simulink model "mymodel_lilio"  (R2017a)
settings: Solver=FixedStepAuto  StartTime=0  StopTime=100  FixedStep=0.05  RelTol=1e-3
settings Model: Creator=bsolv  LastModifiedBy=bsolv

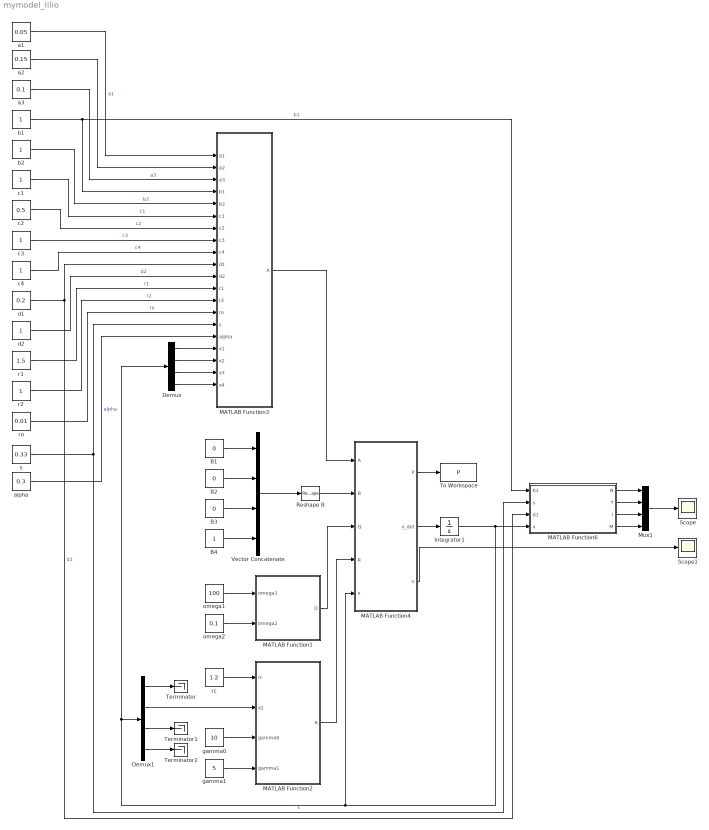
== system mymodel_lilio ==
  B1 : Constant  Value=0
  B2 : Constant  Value=0
  B3 : Constant  Value=0
  B4 : Constant
  Demux : Demux
  Demux1 : Demux
  Integrator1 : Integrator  InitialCondition=[1-1;0.2;0.15-1.65;0]
  MATLAB Function1 : MATLAB Function  TreatAsAtomicUnit=on
  MATLAB Function2 : MATLAB Function  TreatAsAtomicUnit=on
  MATLAB Function3 : MATLAB Function  TreatAsAtomicUnit=on
  MATLAB Function4 : MATLAB Function  TreatAsAtomicUnit=on
  MATLAB Function6 : MATLAB Function  TreatAsAtomicUnit=on
  Mux1 : Mux
  Reshape B : Reshape  OutputDimensionality=Column vector (2-D)
  Scope : Scope
  Scope1 : Scope
  Terminator : Terminator
  Terminator1 : Terminator
  Terminator2 : Terminator
  To Workspace : ToWorkspace  VariableName=P  SampleTime=1
  Vector Concatenate : Concatenate  NumInputs=4
  a1 : Constant  Value=0.05
  a2 : Constant  Value=0.15
  a3 : Constant  Value=0.1
  alpha : Constant  Value=0.3
  b1 : Constant
  b2 : Constant
  c1 : Constant
  c2 : Constant  Value=0.5
  c3 : Constant
  c4 : Constant
  d1 : Constant  Value=0.2
  d2 : Constant
  gamma0 : Constant  Value=10
  gamma1 : Constant  Value=5
  omega1 : Constant  Value=100
  omega2 : Constant  Value=0.1
  r1 : Constant  Value=1.5
  r2 : Constant
  rc : Constant  Value=1.2
  ro : Constant  Value=0.01
  s : Constant  Value=0.33
  wires:
  omega2/1 -> MATLAB Function1/2(omega2)
  omega1/1 -> MATLAB Function1/1(omega1)
  rc/1 -> MATLAB Function2/1(rc)
  gamma0/1 -> MATLAB Function2/3(gamma0)
  B1/1 -> Vector Concatenate/1
  B2/1 -> Vector Concatenate/2
  B3/1 -> Vector Concatenate/3
  B4/1 -> Vector Concatenate/4
  Vector Concatenate/1 -> Reshape B/1
  MATLAB Function3/1(A) -> MATLAB Function4/1(A)
  Reshape B/1 -> MATLAB Function4/2(B)
  MATLAB Function1/1(Q) -> MATLAB Function4/3(Q)
  MATLAB Function2/1(R) -> MATLAB Function4/4(R)
  Demux/1 -> MATLAB Function3/17(x1)
  Demux/2 -> MATLAB Function3/18(x2)
  Demux/3 -> MATLAB Function3/19(x3)
  Demux/4 -> MATLAB Function3/20(x4)
  a1/1 -> MATLAB Function3/1(a1)  "a1"
  a2/1 -> MATLAB Function3/2(a2)
  a3/1 -> MATLAB Function3/3(a3)  "a3"
  b1/1 -> MATLAB Function6/1(b1), MATLAB Function3/4(b1)  "b1"
  b2/1 -> MATLAB Function3/5(b2)  "b2"
  c1/1 -> MATLAB Function3/6(c1)  "c1"
  c2/1 -> MATLAB Function3/7(c2)  "c2"
  c3/1 -> MATLAB Function3/8(c3)  "c3"
  c4/1 -> MATLAB Function3/9(c4)  "c4"
  d1/1 -> MATLAB Function3/10(d1), MATLAB Function6/3(d1)  "d1"
  d2/1 -> MATLAB Function3/11(d2)  "d2"
  r1/1 -> MATLAB Function3/12(r1)  "r1"
  r2/1 -> MATLAB Function3/13(r2)  "r2"
  s/1 -> MATLAB Function3/15(s), MATLAB Function6/2(s)  "s"
  ro/1 -> MATLAB Function3/14(ro)  "ro"
  alpha/1 -> MATLAB Function3/16(alpha)  "alpha"
  MATLAB Function6/1(N) -> Mux1/1
  MATLAB Function6/2(T) -> Mux1/2
  MATLAB Function6/3(I) -> Mux1/3
  MATLAB Function6/4(M) -> Mux1/4
  Demux1/2 -> MATLAB Function2/2(x2)
  MATLAB Function4/2(x_dot) -> Integrator1/1
  Integrator1/1 -> MATLAB Function6/4(x), MATLAB Function4/5(x), Demux/1, Demux1/1
  Demux1/1 -> Terminator/1
  Demux1/3 -> Terminator1/1
  Demux1/4 -> Terminator2/1
  MATLAB Function4/1(P) -> To Workspace/1
  Mux1/1 -> Scope/1
  gamma1/1 -> MATLAB Function2/4(gamma1)
  MATLAB Function4/3(u) -> Scope1/1

== matlab function mymodel_lilio/MATLAB Function1 ==
  data: omega1 input; Q output; omega2 input
function Q = Q_matrix(omega1, omega2)
    Q = [ 0 0 0 0; 
          0 omega1 0 0; 
          0 0 0 0; 
          0 0 0 omega2];

== matlab function mymodel_lilio/MATLAB Function2 ==
  data: rc input; R output; x2 input; gamma0 input; gamma1 input
function R = R_matrix(rc, x2, gamma0, gamma1)

%R = rc +gamma0*x2;
%R = rc -gamma1*x2;
R = rc;

== matlab function mymodel_lilio/MATLAB Function3 ==
  data: a1 input; A output; a2 input; a3 input; b1 input; b2 input; c1 input; c2 input; c3 input; c4 input; d1 input; d2 input; r1 input; r2 input; ro input; s input; alpha input; x1 input; x2 input; x3 input; x4 input
function A = A_matrix(a1, a2, a3, b1, b2, c1, c2, c3, c4, d1, d2, r1, r2, ro, s, alpha, x1, x2, x3, x4)

    A11 =  -r2*(1+b2*x1);
    A12 =  -c4*(x1 + 1/b2);
    A13 =  0;
    A14 =  -a1*(1/b2 + x1);

    A21 =  -c3*x2;
    A22 =  r1*(1-b1*x2)-(c2*s/d1 + c3/b2);
    A23 =  -c2*x2;
    A24 =  -a2*x2;

    A31 =  0;
    A32 =  ro*(x3 + s/d1)/(alpha + x2) -c1*(x3+s/d1) -x4;
    A33 =  -d1;
    A34 =  -a3*(x3 +s/d1)+x2;

    A41 =  0;
    A42 =  0;
    A43 =  0;
    A44 =  -d2;
    
    A = [A11 A12 A13 A14;
         A21 A22 A23 A24;
         A31 A32 A33 A34;
         A41 A42 A43 A44];

== matlab function mymodel_lilio/MATLAB Function4 ==
  data: P output; A input; B input; Q input; R input; x input; x_dot output; u output
function [P, x_dot, u] = SDRE(A, B, Q, R, x)

coder.extrinsic('lqr');
coder.extrinsic('dlqr');
coder.extrinsic('lqrd');
coder.extrinsic('care');
coder.extrinsic('dare');
coder.extrinsic('eig');
coder.extrinsic('rank');
coder.extrinsic('size');
coder.extrinsic('chol');
coder.extrinsic('all');
coder.extrinsic('eps');
coder.extrinsic('inv');

control = 1;
bound = 0;

u = 0;
u_min = 0;
u_max = 1;
P = zeros(4,4);
x_dot = zeros(4,1);


if(control)
    L = zeros(4,1);
    G = zeros(1,4);
    S = zeros(4,1);
    E = eye(4);
    
    M=[B A*B (A^2)*B (A^3)*B];
    rankM=rank(M);
    
    %[P,~,G] = care(A,B,Q,R,S,E);
    P = ARE_diag(A, B, Q, R);
    G = (R\B')*P;
    u_unb = -G*x;
    
    if(bound)
        u = min(max(u_unb,u_min),u_max);
    else
        u = u_unb;
    end
    
    %x_dot = (A-B*G)*x;
    x_dot = (A*x+B*u);
else
    u = 0;
    x_dot = (A)*x;
end

== matlab function mymodel_lilio/MATLAB Function6 ==
  data: b1 input; s input; d1 input; x input; N output; T output; I output; M output
function [N, T, I, M] = DimensionaliseModel(b1, s, d1, x)

N = 0;
T = 0;
I = 0;
M = 0;

N = x(1) + 1/b1;
T = x(2);
I = x(3) + s/d1;
M = x(4);
